simulink model "ekf_djax_1"  (R2013a)
settings: Solver=ode45  StartTime=0.0  StopTime=10.0  RelTol=1e-3
values from neighbouring files (symbols this model uses):
  A = [0, 1; 0, 0]    [run_ekf.m]
  B = [0;1]    [run_ekf.m]
  C = [1,0]    [run_ekf.m]
  P0_guess = [0,0;0, 15]    [run_ekf.m]
  Q = 0.05*eye(2)    [run_ekf.m]
  R = 0.5    [run_ekf.m]
  x0_guess = [0;15]    [run_ekf.m]
settings Model: Creator=DJackson  LastModifiedBy=DJackson

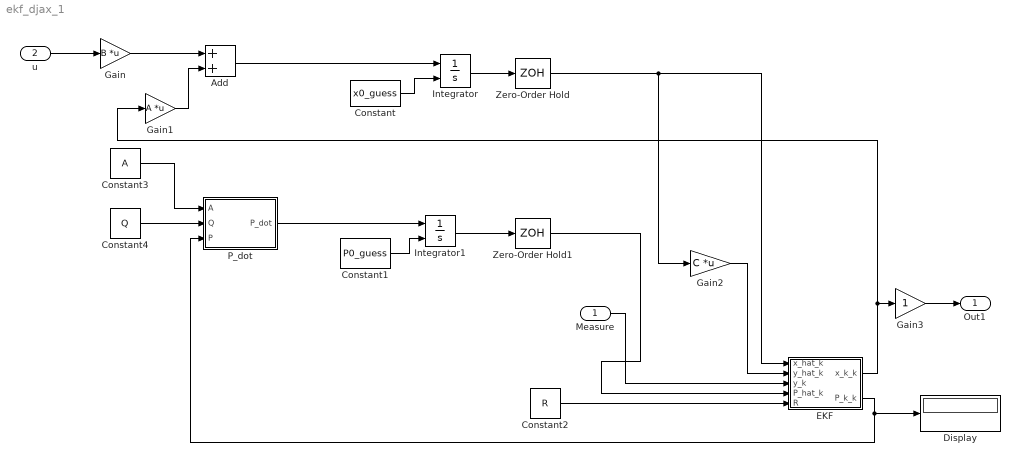
== system ekf_djax_1 ==
  Measure : Inport
  u : Inport  Port=2
  Add : Sum
  Constant : Constant  Value=x0_guess
  Constant1 : Constant  Value=P0_guess
  Constant2 : Constant  Value=R
  Constant3 : Constant  Value=A
  Constant4 : Constant  Value=Q
  Display : Display
  EKF : MATLAB Function  TreatAsAtomicUnit=on
  Gain : Gain  Gain=B  Multiplication=Matrix(K*u)
  Gain1 : Gain  Gain=A  Multiplication=Matrix(K*u)
  Gain2 : Gain  Gain=C  Multiplication=Matrix(K*u)
  Gain3 : Gain
  Integrator : Integrator  InitialConditionSource=external
  Integrator1 : Integrator  InitialConditionSource=external
  P_dot : MATLAB Function  TreatAsAtomicUnit=on
  Zero-Order Hold : ZeroOrderHold
  Zero-Order Hold1 : ZeroOrderHold
  Out1 : Outport
  wires:
  u/1 -> Gain/1
  Gain/1 -> Add/1
  Gain1/1 -> Add/2
  Add/1 -> Integrator/1
  Integrator/1 -> Zero-Order Hold/1
  Constant/1 -> Integrator/2
  Gain2/1 -> EKF/2(y_hat_k)
  Measure/1 -> EKF/3(y_k)
  Constant2/1 -> EKF/5(R)
  Zero-Order Hold1/1 -> EKF/4(P_hat_k)
  Integrator1/1 -> Zero-Order Hold1/1
  Constant1/1 -> Integrator1/2
  Zero-Order Hold/1 -> Gain2/1, EKF/1(x_hat_k)
  P_dot/1(P_dot) -> Integrator1/1
  Constant3/1 -> P_dot/1(A)
  Constant4/1 -> P_dot/2(Q)
  EKF/2(P_k_k) -> P_dot/3(P), Display/1
  Gain3/1 -> Out1/1
  EKF/1(x_k_k) -> Gain1/1, Gain3/1

== matlab function ekf_djax_1/P_dot ==
  data: A input; P_dot output; Q input; P input
function P_dot = fcn(A,Q,P)
%#coder

P_dot = A*P + P*A' + Q;

== matlab function ekf_djax_1/EKF ==
  data: x_hat_k input; x_k_k output; y_hat_k input; y_k input; P_hat_k input; R input; P_k_k output
function [x_k_k, P_k_k] = fcn(x_hat_k , y_hat_k, y_k  ,P_hat_k,R)
%#coder
C = [1 0];

K = P_hat_k*C'*inv(C*P_hat_k*C' + R); %Kalman gain

x_k_k = x_hat_k + K*(y_k - y_hat_k); %Correction step for time 'k'
P_k_k = (eye(2) - K*C)*P_hat_k*(eye(2) - K*C)' + K*R*K'; % Covariance matrix update
